simulink model "Ungekoppelt_Plot"  (R2019b)
settings: Solver=VariableStepAuto  StartTime=0.0  StopTime=200  RelTol=1e-3
undefined symbols (not defined in the file): A1, A2, A3, k1, k2, k3, Kv
libraries: simulink x1
settings Model: OrderedModelArguments=off  Creator=Ogulcan  LastModifiedBy=Ogulcan

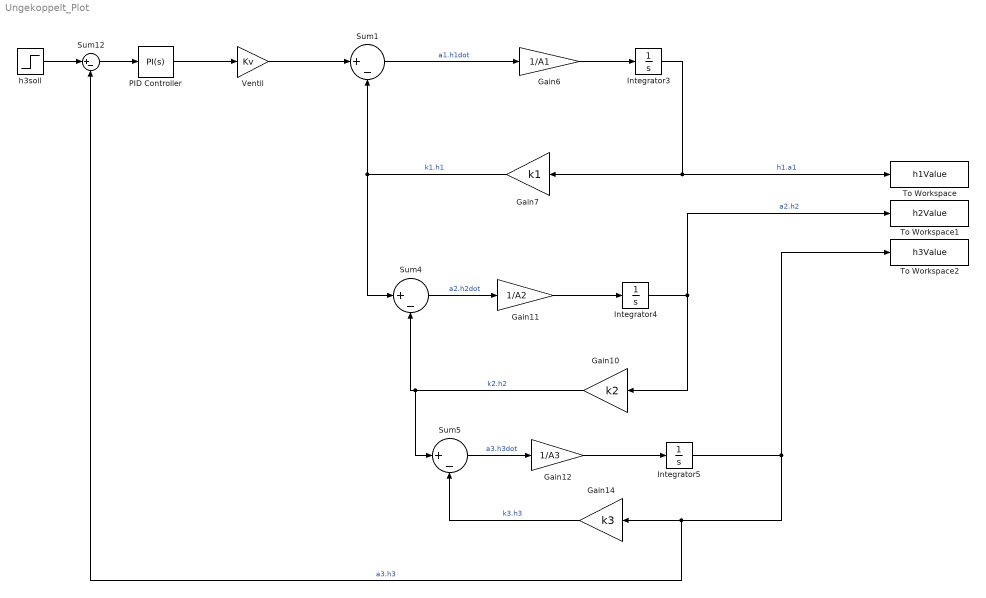
== system Ungekoppelt_Plot ==
  Gain10 : Gain  Gain=k2
  Gain11 : Gain  Gain=1/A2
  Gain12 : Gain  Gain=1/A3
  Gain14 : Gain  Gain=k3
  Gain6 : Gain  Gain=1/A1
  Gain7 : Gain  Gain=k1
  Integrator3 : Integrator
  Integrator4 : Integrator
  Integrator5 : Integrator
  PID Controller : simulink/Continuous/PID Controller  Controller=PI  Form=Ideal  TimeDomain=Continuous-time  SampleTime=-1  IntegratorMethod=Forward Euler  FilterMethod=Forward Euler  ControllerParametersSource=internal  P=0.1  I=0.05  D=0  UseFilter=on  N=100  TunerSelectOption=Transfer Function Based (PID Tuner App)  InitialConditionSource=internal  InitialConditionForIntegrator=0  InitialConditionForFilter=0  DifferentiatorICPrevScaledInput=0  ExternalReset=none  TrackingMode=off  Kt=1  LimitOutput=off  UpperSaturationLimit=inf  LowerSaturationLimit=-inf  LinearizeAsGain=on  AntiWindupMode=none  Kb=1  POutMin=[]  POutMax=[]  IOutMin=[]  IOutMax=[]  DOutMin=[]  DOutMax=[]  NOutMin=[]  NOutMax=[]  SumOutMin=[]  SumOutMax=[]  SaturationOutMin=[]  SaturationOutMax=[]  PParamMin=[]  PParamMax=[]  IParamMin=[]  IParamMax=[]  DParamMin=[]  DParamMax=[]  NParamMin=[]  NParamMax=[]  KbParamMin=[]  KbParamMax=[]  KtParamMin=[]  KtParamMax=[]  KbOutMin=[]  KbOutMax=[]  KtOutMin=[]  KtOutMax=[]  IntegratorOutMin=[]  IntegratorOutMax=[]  FilterOutMin=[]  FilterOutMax=[]  SumI1OutMin=[]  SumI1OutMax=[]  SumI2OutMin=[]  SumI2OutMax=[]  SumI3OutMin=[]  SumI3OutMax=[]  SumI4OutMin=[]  SumI4OutMax=[]  SumDOutMin=[]  SumDOutMax=[]  DifferentiatorOutMin=[]  DifferentiatorOutMax=[]  FilterDiffOutCoefMin=[]  FilterDiffOutCoefMax=[]  ReciprocalOutMin=[]  ReciprocalOutMax=[]  SumDenOutMin=[]  SumDenOutMax=[]  SumNumOutMin=[]  SumNumOutMax=[]  DivideOutMin=[]  DivideOutMax=[]  IntegratorContinuousStateAttributes=''  IntegratorStateMustResolveToSignalObject=off  IntegratorRTWStateStorageClass=Auto  FilterContinuousStateAttributes=''  FilterStateMustResolveToSignalObject=off  FilterRTWStateStorageClass=Auto  ParallelPVariant=Passthrough  IdealPVariant=InternalParameters  IVariant=InternalParameters  DVariant=Disabled  IntegratorVariant=Continuous  SatVariant=Disabled  AWVariant=Passthrough  PCopyVariant=Disabled  TRVariant=Disabled  FdbkBlocksVariant=Forward  IdealPFdbkVariant=Disabled  SatFdbkVariant=Disabled  DerivativeFilterVariant=Disabled  NVariant=Disabled  NCopyVariant=Disabled_SignalSpec  FilterICVariant=Disabled  IntegratorICVariant=InternalICs  ExternalResetVariant=Disabled  TRSumVariant=Passthrough  SumFdbkVariant=Disabled  SumVariant=Sum_PI
  Sum{1,4..5,12} (4 alike) : Sum  Inputs=|+-
  To Workspace : ToWorkspace  VariableName=h1Value  SaveFormat=Timeseries  SampleTime=-1
  To Workspace1 : ToWorkspace  VariableName=h2Value  SaveFormat=Timeseries  SampleTime=-1
  To Workspace2 : ToWorkspace  VariableName=h3Value  SaveFormat=Timeseries  SampleTime=-1
  Ventil : Gain  Gain=Kv
  h3soll : Step  After=100  SampleTime=0
  wires:
  Integrator3/1 -> To Workspace/1, Gain7/1  "h1.a1"
  Gain7/1 -> Sum4/1, Sum1/2  "k1.h1"
  Integrator4/1 -> To Workspace1/1, Gain10/1  "a2.h2"
  Gain10/1 -> Sum5/1, Sum4/2  "k2.h2"
  Integrator5/1 -> To Workspace2/1, Gain14/1, Sum12/2  "a3.h3"
  Gain14/1 -> Sum5/2  "k3.h3"
  Sum12/1 -> PID Controller/1
  PID Controller/1 -> Ventil/1
  Sum1/1 -> Gain6/1  "a1.h1dot"
  Gain6/1 -> Integrator3/1
  h3soll/1 -> Sum12/1
  Gain11/1 -> Integrator4/1
  Sum4/1 -> Gain11/1  "a2.h2dot"
  Gain12/1 -> Integrator5/1
  Sum5/1 -> Gain12/1  "a3.h3dot"
  Ventil/1 -> Sum1/1
